simulink model "encoder_parametro_Nr"  (R2012b)
settings: Solver=ode3  StartTime=0.0  StopTime=6  FixedStep=1e-4  RelTol=1e-6
libraries: simulink x1
settings Model: Creator=Juliano  LastModifiedBy=Juliano

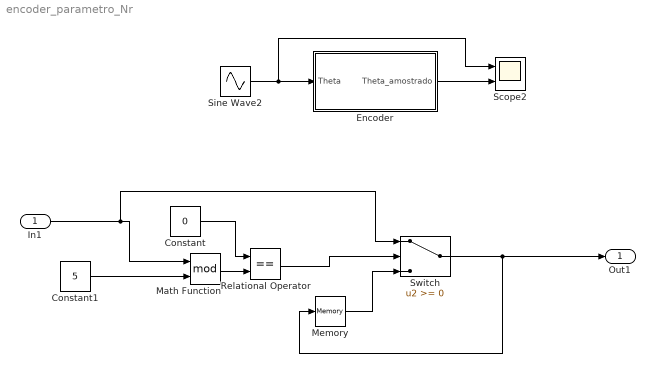
== system encoder_parametro_Nr ==
  In1 : Inport
  Constant : Constant  Value=0
  Constant1 : Constant  Value=5
  Encoder : Subsystem  mask{Nr=72}
      mask prompts: Nr "Número de pulsos por revolução"
  Math Function : Math  Operator=mod  SaturateOnIntegerOverflow=on
  Memory : Memory
  Relational Operator : RelationalOperator  Operator===  OutDataTypeStr=boolean
  Scope2 : Scope  NumInputPorts=2
      settings: YMin=150~0  YMax=575~375
  Sine Wave2 : Sin  Amplitude=360  SampleTime=0
  Switch : Switch
  Out1 : Outport
  wires:
  Encoder/1(Theta_amostrado) -> Scope2/2
  Sine Wave2/1 -> Scope2/1, Encoder/1(Theta)
  In1/1 -> Switch/1, Math Function/1
  Switch/1 -> Out1/1, Memory/1
  Math Function/1 -> Relational Operator/2
  Relational Operator/1 -> Switch/2
  Constant/1 -> Relational Operator/1
  Constant1/1 -> Math Function/2
  Memory/1 -> Switch/3

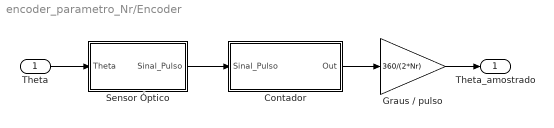
== system encoder_parametro_Nr/Encoder ==
  Theta : Inport
  Contador : Subsystem
  Graus / pulso : Gain  Gain=360/(2*Nr)
  Sensor Óptico : Subsystem
  Theta_amostrado : Outport
  wires:
  Contador/1(Out) -> Graus / pulso/1
  Sensor Óptico/1(Sinal_Pulso) -> Contador/1(Sinal_Pulso)
  Theta/1 -> Sensor Óptico/1(Theta)
  Graus / pulso/1 -> Theta_amostrado/1

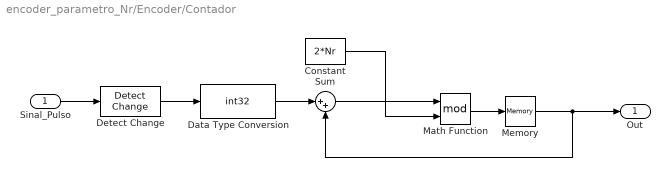
== system encoder_parametro_Nr/Encoder/Contador ==
  Sinal_Pulso : Inport
  Constant : Constant  Value=2*Nr
  Data Type Conversion : DataTypeConversion  OutDataTypeStr=int32
  Detect Change : simulink/Logic and Bit Operations/Detect Change  vinit=0  InputProcessing=Inherited  OutDataTypeStr=boolean
  Math Function : Math  Operator=mod  SaturateOnIntegerOverflow=on
  Memory : Memory
  Sum : Sum  Inputs=|++
  Out : Outport
  wires:
  Sinal_Pulso/1 -> Detect Change/1
  Memory/1 -> Out/1, Sum/2
  Constant/1 -> Math Function/2
  Detect Change/1 -> Data Type Conversion/1
  Data Type Conversion/1 -> Sum/1
  Math Function/1 -> Memory/1
  Sum/1 -> Math Function/1

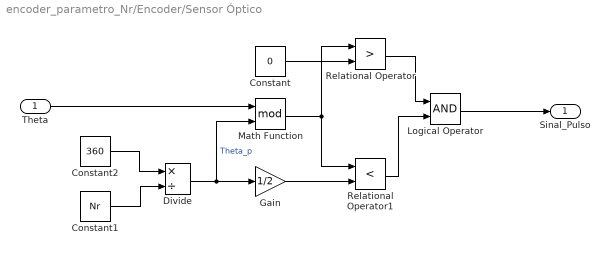
== system encoder_parametro_Nr/Encoder/Sensor Óptico ==
  Theta : Inport
  Constant : Constant  Value=0
  Constant1 : Constant  Value=Nr
  Constant2 : Constant  Value=360
  Divide : Product  Inputs=*/
  Gain : Gain  Gain=1/2
  Logical Operator : Logic  AllPortsSameDT=off  OutDataTypeStr=boolean
  Math Function : Math  Operator=mod  SaturateOnIntegerOverflow=on
  Relational Operator : RelationalOperator  Operator=>  OutDataTypeStr=boolean
  Relational Operator1 : RelationalOperator  Operator=<  OutDataTypeStr=boolean
  Sinal_Pulso : Outport
  wires:
  Math Function/1 -> Relational Operator1/1, Relational Operator/1
  Theta/1 -> Math Function/1
  Relational Operator/1 -> Logical Operator/1
  Relational Operator1/1 -> Logical Operator/2
  Constant/1 -> Relational Operator/2
  Divide/1 -> Math Function/2, Gain/1  "Theta_p"
  Gain/1 -> Relational Operator1/2
  Logical Operator/1 -> Sinal_Pulso/1
  Constant2/1 -> Divide/1
  Constant1/1 -> Divide/2
